simulink model "sampleModel1466"  (R2023a)
settings: Solver=VariableStepAuto  StartTime=0.0  StopTime=10.0  RelTol=1e-3
libraries: hdlsllib x3, simulink x1
settings Model: Creator=user1  LastModifiedBy=user1

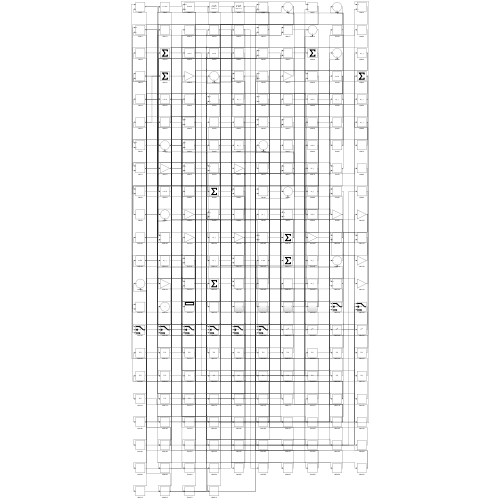
[thumbnail: Simulink's stored preview of the top-level diagram]
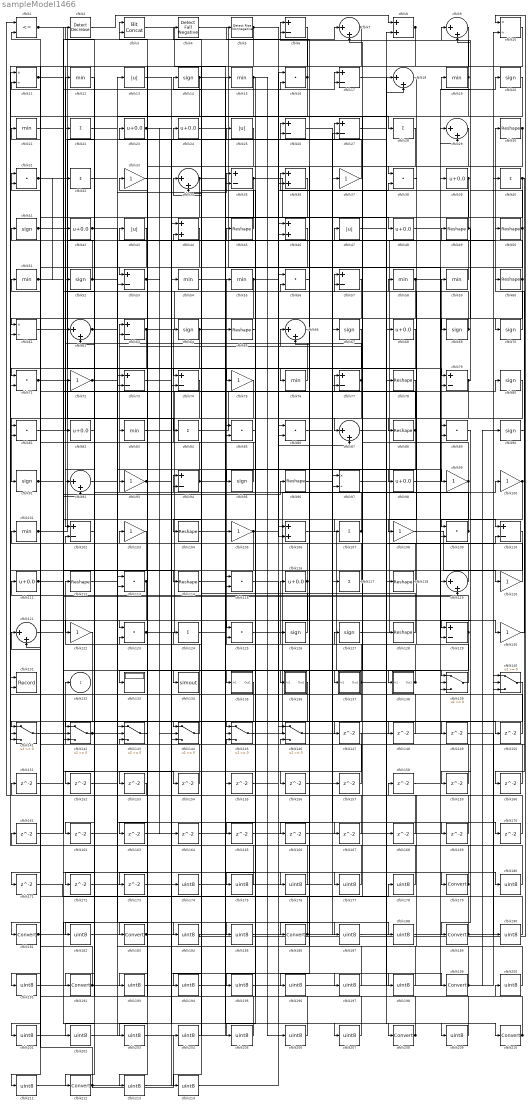
== system sampleModel1466 ==
  cfblk1 : RelationalOperator  Operator=<=  OutDataTypeStr=boolean  InputSameDT=off
  cfblk{10..11,61,97} (4 alike) : Product  Inputs=*/  RndMeth=Zero  SaturateOnIntegerOverflow=on
  cfblk{33,37,72,75,93,99..100,103,105,108,120,122,130} (13 alike) : Gain
  cfblk{12,15,19,21,51,54..55,58..59,76,83,101} (12 alike) : MinMax
  cfblk{6,17,26..27,35,53,57,63,73..74,77,79,94,102,110,129} (16 alike) : Sum  Inputs=+-
  cfblk{30,45,49..50,60,65,78,88,96,104,112,114,118,128} (14 alike) : Reshape
  cfblk{8,36,44,46,106} (5 alike) : Sum
  cfblk{22,28,32,40,84,107,117,124} (8 alike) : Sum  Inputs=+
  cfblk{16,31,38,56,71,81,85..86,89,109,113,115,123,125} (14 alike) : DotProduct  OutDataTypeStr=Inherit: Inherit via internal rule
  cfblk{23..24,39,42,48,68,82,98,111,116} (10 alike) : Bias  Bias=0.0  SaturateOnIntegerOverflow=off
  cfblk{7,9,18,29,34,62,66,87,92,119,121} (11 alike) : Sum  Inputs=|++
  cfblk{14,20,41,52,64,67,69..70,80,90..91,95,126..127} (14 alike) : Signum
  cfblk{13,25,43,47} (4 alike) : Abs  SaturateOnIntegerOverflow=off
  cfblk131 : Record  FileSettingsInternal="{\"entries\":[{\"content\":{\"excelSettings\":{\"content\":{},\"type\":\"Streamout.ExcelSettings\"}},\"type\":\"Streamout.FileSettingStorage\",\"uuid\":\"\"}],\"packageUris\":[\"http:\\/\\/schema.mathworks.com\\/mf0\\/streamout_blocks\\/R2020a\"],\"version\":\"1.0\"}"  Layout=[1 1]  SignalsInternal="{\"entries\":[{\"content\":{\"signals\":[{\"content\":{\"blockPath\":[],\"dimensions\":[1],\"domain\":\"\",\"lineColor\":\"#a2142f\",\"plots\":[1],\"port\":1,\"signalID\":882,\"signalName\":\"XY Graph:1\"},\"type\":\"RecordBlkView.Signal\",\"uuid\":\"\"},{\"content\":{\"blockPath\":[],\"dimensions\":[1],\"domain\":\"\",\"lineColor\":\"#139fff\",\"plots\":[1],\"port\":2,\"signalID\":885,\"signalName\":\"XY Graph:2\"},\"type\":\"RecordBlkView.Signal\",\"uuid\":\"\"}]},\"type\":\"RecordBlkView.InputSignals\",\"uuid\":\"\"}],\"packageUris\":[\"http:\\/\\/schema.mathworks.com\\/mf0\\/streamout_blocks\\/R2020a\"],\"version\":\"1.0\"}"  VisualizationBindings="{\"xyplotplugin\":{\"info\":[{\"series\":[{\"bindingParametersList\":[{\"parameter\":\"X-Axis\",\"signalID\":882,\"signalName\":\"XY Graph:1\"},{\"parameter\":\"Y-Axis\",\"signalID\":885,\"signalName\":\"XY Graph:2\"}],\"seriesID\":5313}],\"subplotID\":1}]}}"  CompatibilityTag=XY  st=-1
  cfblk133 : Display
  cfblk134 : ToWorkspace  VariableName=simout  SaveFormat=Timeseries  SampleTime=-1
  cfblk135 : Subsystem
      settings: LibrarySourceBlock=|
      | hdlsllib/Ports &
      | Subsystems/Subsystem
  cfblk136 : Subsystem
      settings: LibrarySourceBlock=|
      | hdlsllib/Ports &
      | Subsystems/Subsystem
  cfblk137 : Subsystem
      settings: LibrarySourceBlock=|
      | hdlsllib/Ports &
      | Subsystems/Subsystem
  cfblk138 : Subsystem
      settings: LibrarySourceBlock=|
      | hdlsllib/Ports &
      | Subsystems/Subsystem
  cfblk{139..146} (8 alike) : Switch  SaturateOnIntegerOverflow=off  InputSameDT=off
  cfblk{147..173} (27 alike) : Delay  SampleTime=1
  cfblk{174..178,180,182,184..185,187..188,190..191,193..198,200..207,209,211,213..214} (31 alike) : DataTypeConversion  OutDataTypeStr=uint8  SaturateOnIntegerOverflow=off  RndMeth=Floor
  cfblk{179,181,183,186,189,192,199,208,210,212} (10 alike) : DataTypeConversion  SaturateOnIntegerOverflow=off  RndMeth=Floor
  cfblk2 : simulink/Logic and Bit Operations/Detect Decrease  vinit=0.0  OutDataTypeStr=boolean
      settings: LibrarySourceBlock=|
      | hdlsllib/Logic and Bit
      | Operations/Detect
      | Decrease
  cfblk3 : hdlsllib/Logic and Bit Operations/Bit Concat  numInputs=2
  cfblk4 : hdlsllib/Logic and Bit Operations/Detect Fall Negative  vinit=0  OutDataTypeStr=boolean
  cfblk5 : hdlsllib/Logic and Bit Operations/Detect Rise Nonnegative  vinit=0  OutDataTypeStr=boolean
  cfblk132 : Outport  VectorParamsAs1DForOutWhenUnconnected=off
  wires:
  cfblk70/1 -> cfblk30/1
  cfblk123/1 -> cfblk80/1, cfblk197/1
  cfblk23/1 -> cfblk144/2, cfblk177/1
  cfblk31/1 -> cfblk26/1, cfblk180/1
  cfblk126/1 -> cfblk14/1
  cfblk98/1 -> cfblk59/1
  cfblk41/1 -> cfblk18/1, cfblk136/1(In1), cfblk147/1
  cfblk138/1(Out1) -> cfblk55/1, cfblk126/1, cfblk57/2
  cfblk127/1 -> cfblk50/1
  cfblk124/1 -> cfblk179/1
  cfblk106/1 -> cfblk138/1(In1)
  cfblk45/1 -> cfblk23/1
  cfblk145/1 -> cfblk100/1
  cfblk19/1 -> cfblk6/1, cfblk87/1
  cfblk101/1 -> cfblk49/1, cfblk92/2
  cfblk144/1 -> cfblk112/1
  cfblk139/1 -> cfblk58/1
  cfblk69/1 -> cfblk19/1, cfblk7/2
  cfblk90/1 -> cfblk132/1
  cfblk48/1 -> cfblk20/1
  cfblk18/1 -> cfblk108/1
  cfblk4/1 -> cfblk119/1
  cfblk79/1 -> cfblk122/1, cfblk9/1
  cfblk76/1 -> cfblk65/1
  cfblk61/1 -> cfblk27/1
  cfblk13/1 -> cfblk145/1
  cfblk3/1 -> cfblk115/1
  cfblk104/1 -> cfblk105/1
  cfblk120/1 -> cfblk101/1
  cfblk97/1 -> cfblk68/1
  cfblk36/1 -> cfblk95/1
  cfblk100/1 -> cfblk129/1, cfblk159/1
  cfblk83/1 -> cfblk208/1
  cfblk5/1 -> cfblk102/1, cfblk87/2
  cfblk125/1 -> cfblk130/1
  cfblk8/1 -> cfblk104/1, cfblk81/2
  cfblk109/1 -> cfblk63/1, cfblk2/1
  cfblk1/1 -> cfblk75/1, cfblk207/1
  cfblk59/1 -> cfblk3/1
  cfblk49/1 -> cfblk69/1, cfblk6/2
  cfblk29/1 -> cfblk186/1
  cfblk140/1 -> cfblk192/1
  cfblk64/1 -> cfblk97/2, cfblk141/2
  cfblk142/1 -> cfblk144/1, cfblk184/1
  cfblk81/1 -> cfblk12/1
  cfblk77/1 -> cfblk62/1, cfblk125/2
  cfblk25/1 -> cfblk123/1
  cfblk62/1 -> cfblk35/1, cfblk26/2, cfblk135/1(In1)
  cfblk7/1 -> cfblk53/1, cfblk81/1
  cfblk143/1 -> cfblk103/1
  cfblk58/1 -> cfblk39/1, cfblk82/1
  cfblk63/1 -> cfblk57/1, cfblk162/1
  cfblk88/1 -> cfblk21/1, cfblk195/1
  cfblk107/1 -> cfblk45/1, cfblk42/1
  cfblk95/1 -> cfblk64/1
  cfblk22/1 -> cfblk28/1
  cfblk12/1 -> cfblk92/1
  cfblk129/1 -> cfblk111/1, cfblk203/1
  cfblk46/1 -> cfblk212/1
  cfblk118/1 -> cfblk36/1
  cfblk15/1 -> cfblk125/1, cfblk152/1, cfblk206/1
  cfblk99/1 -> cfblk129/2, cfblk63/2
  cfblk102/1 -> cfblk22/1
  cfblk11/1 -> cfblk114/1, cfblk119/2
  cfblk34/1 -> cfblk48/1, cfblk191/1
  cfblk146/1 -> cfblk40/1
  cfblk108/1 -> cfblk120/1
  cfblk2/1 -> cfblk8/1
  cfblk113/1 -> cfblk142/1, cfblk142/3, cfblk171/1
  cfblk74/1 -> cfblk131/2
  cfblk9/1 -> cfblk74/1
  cfblk42/1 -> cfblk143/1, cfblk99/1
  cfblk55/1 -> cfblk143/2, cfblk38/2
  cfblk37/1 -> cfblk4/1
  cfblk75/1 -> cfblk91/1
  cfblk10/1 -> cfblk183/1
  cfblk54/1 -> cfblk210/1
  cfblk60/1 -> cfblk70/1, cfblk3/2, cfblk71/2
  cfblk110/1 -> cfblk134/1
  cfblk128/1 -> cfblk24/1
  cfblk117/1 -> cfblk94/1
  cfblk93/1 -> cfblk25/1, cfblk198/1
  cfblk51/1 -> cfblk32/1, cfblk149/1
  cfblk35/1 -> cfblk118/1, cfblk201/1
  cfblk43/1 -> cfblk71/1
  cfblk16/1 -> cfblk5/1, cfblk61/2
  cfblk6/1 -> cfblk34/2
  cfblk94/1 -> cfblk11/2, cfblk139/1
  cfblk114/1 -> cfblk77/1
  cfblk50/1 -> cfblk106/2, cfblk9/2
  cfblk71/1 -> cfblk84/1, cfblk56/2
  cfblk78/1 -> cfblk181/1
  cfblk72/1 -> cfblk13/1, cfblk17/2
  cfblk52/1 -> cfblk31/1, cfblk167/1
  cfblk39/1 -> cfblk137/1(In1), cfblk98/1, cfblk166/1
  cfblk135/1(Out1) -> cfblk141/1
  cfblk53/1 -> cfblk163/1, cfblk164/1
  cfblk32/1 -> cfblk17/1
  cfblk24/1 -> cfblk109/1
  cfblk119/1 -> cfblk93/1
  cfblk40/1 -> cfblk72/1, cfblk160/1
  cfblk14/1 -> cfblk79/1, cfblk172/1
  cfblk84/1 -> cfblk67/1
  cfblk89/1 -> cfblk189/1
  cfblk111/1 -> cfblk96/1, cfblk79/2
  cfblk73/1 -> cfblk199/1
  cfblk92/1 -> cfblk53/2
  cfblk116/1 -> cfblk43/1, cfblk133/1
  cfblk20/1 -> cfblk74/2
  cfblk47/1 -> cfblk110/1
  cfblk30/1 -> cfblk38/1, cfblk76/1
  cfblk57/1 -> cfblk61/1
  cfblk91/1 -> cfblk107/1, cfblk16/2
  cfblk86/1 -> cfblk117/1
  cfblk105/1 -> cfblk47/1, cfblk141/3
  cfblk38/1 -> cfblk88/1
  cfblk82/1 -> cfblk52/1
  cfblk141/1 -> cfblk7/1
  cfblk137/1(Out1) -> cfblk116/1, cfblk110/2, cfblk165/1
  cfblk130/1 -> cfblk60/1
  cfblk115/1 -> cfblk148/1
  cfblk148/1 -> cfblk11/1
  cfblk17/1 -> cfblk150/1
  cfblk150/1 -> cfblk34/1
  cfblk152/1 -> cfblk113/2
  cfblk28/1 -> cfblk153/1
  cfblk153/1 -> cfblk1/1
  cfblk21/1 -> cfblk154/1
  cfblk154/1 -> cfblk62/2
  cfblk155/1 -> cfblk86/2
  cfblk56/1 -> cfblk156/1
  cfblk156/1 -> cfblk27/2
  cfblk96/1 -> cfblk157/1
  cfblk157/1 -> cfblk145/2
  cfblk158/1 -> cfblk109/2
  cfblk159/1 -> cfblk1/2
  cfblk160/1 -> cfblk123/2
  cfblk161/1 -> cfblk142/2
  cfblk163/1 -> cfblk77/2
  cfblk164/1 -> cfblk8/2
  cfblk165/1 -> cfblk18/2
  cfblk166/1 -> cfblk139/3
  cfblk167/1 -> cfblk143/3
  cfblk87/1 -> cfblk168/1
  cfblk168/1 -> cfblk94/2
  cfblk26/1 -> cfblk169/1
  cfblk169/1 -> cfblk35/2
  cfblk112/1 -> cfblk170/1
  cfblk170/1 -> cfblk106/1
  cfblk172/1 -> cfblk36/2
  cfblk136/1(Out1) -> cfblk173/1
  cfblk173/1 -> cfblk97/1
  cfblk33/1 -> cfblk174/1
  cfblk174/1 -> cfblk155/1
  cfblk65/1 -> cfblk175/1
  cfblk175/1 -> cfblk33/1
  cfblk121/1 -> cfblk176/1
  cfblk176/1 -> cfblk86/1
  cfblk177/1 -> cfblk121/1
  cfblk171/1 -> cfblk178/1
  cfblk178/1 -> cfblk121/2
  cfblk179/1 -> cfblk16/1, cfblk145/3, cfblk131/1
  cfblk180/1 -> cfblk124/1
  cfblk181/1 -> cfblk115/2, cfblk187/1
  cfblk103/1 -> cfblk182/1
  cfblk182/1 -> cfblk78/1
  cfblk183/1 -> cfblk139/2, cfblk37/1
  cfblk184/1 -> cfblk10/1
  cfblk162/1 -> cfblk185/1
  cfblk185/1 -> cfblk10/2
  cfblk186/1 -> cfblk146/3, cfblk113/1
  cfblk187/1 -> cfblk29/1
  cfblk151/1 -> cfblk188/1
  cfblk188/1 -> cfblk29/2
  cfblk189/1 -> cfblk31/2, cfblk146/2, cfblk127/1
  cfblk149/1 -> cfblk190/1
  cfblk190/1 -> cfblk89/1
  cfblk191/1 -> cfblk89/2
  cfblk192/1 -> cfblk151/1, cfblk51/1
  cfblk80/1 -> cfblk193/1
  cfblk193/1 -> cfblk140/1
  cfblk67/1 -> cfblk194/1
  cfblk194/1 -> cfblk140/2
  cfblk195/1 -> cfblk140/3
  cfblk66/1 -> cfblk196/1
  cfblk196/1 -> cfblk128/1
  cfblk197/1 -> cfblk66/1
  cfblk198/1 -> cfblk66/2
  cfblk199/1 -> cfblk158/1, cfblk90/1
  cfblk200/1 -> cfblk73/1
  cfblk201/1 -> cfblk73/2
  cfblk44/1 -> cfblk202/1
  cfblk202/1 -> cfblk15/1
  cfblk203/1 -> cfblk44/1
  cfblk204/1 -> cfblk44/2
  cfblk85/1 -> cfblk205/1
  cfblk205/1 -> cfblk102/2
  cfblk206/1 -> cfblk85/1
  cfblk207/1 -> cfblk85/2
  cfblk208/1 -> cfblk161/1, cfblk146/1
  cfblk27/1 -> cfblk209/1
  cfblk209/1 -> cfblk83/1
  cfblk210/1 -> cfblk200/1, cfblk56/1
  cfblk122/1 -> cfblk211/1
  cfblk211/1 -> cfblk54/1
  cfblk212/1 -> cfblk204/1, cfblk144/3, cfblk41/1
  cfblk147/1 -> cfblk213/1
  cfblk213/1 -> cfblk46/1
  cfblk68/1 -> cfblk214/1
  cfblk214/1 -> cfblk46/2

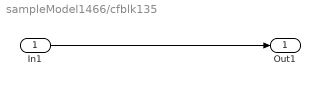
== system sampleModel1466/cfblk135 ==
  In1 : Inport
  Out1 : Outport
  wires:
  In1/1 -> Out1/1

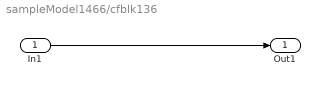
== system sampleModel1466/cfblk136 ==
  In1 : Inport
  Out1 : Outport
  wires:
  In1/1 -> Out1/1

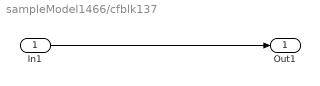
== system sampleModel1466/cfblk137 ==
  In1 : Inport
  Out1 : Outport
  wires:
  In1/1 -> Out1/1

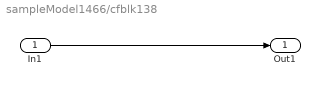
== system sampleModel1466/cfblk138 ==
  In1 : Inport
  Out1 : Outport
  wires:
  In1/1 -> Out1/1
